simulink model "V_Cal"  (R2024b)
settings: Solver=FixedStepAuto  StartTime=0.0  StopTime=inf  RelTol=1e-3  EnableMultiTasking=on
libraries: stm32f4xxblockslib x1
settings Model: STM32="{\"AnalogInput\":[{\"ID\":\"untitled:1\"},{\"ID\":\"V_Cal:1\"}]}"  Creator=jirat  LastModifiedBy=jirat
settings OptimizationCC: DefaultParameterBehavior=Inlined  EnhancedBackFolding=on  PassReuseOutputArgsAs=Individual arguments  ZeroExternalMemoryAtStartup=off  ZeroInternalMemoryAtStartup=off  MaxStackSize=512  OptimizeBlockOrder=speed  DifferentSizesBufferReuse=on  OptimizationCustomize=off  EfficientTunableParamExpr=on
settings DebuggingCC: ParameterTunabilityLossMsg=error
settings HardwareCC: ProdBitPerPointer=32  ProdBitPerSizeT=32  ProdBitPerPtrDiffT=32  ProdLargestAtomicInteger=Long  ProdLargestAtomicFloat=Double  ProdWordSize=32  ProdLongLongMode=on  ProdHWDeviceType=ARM Compatible->ARM Cortex-M
settings SFSimCC: MATLABDynamicMemAlloc=off
settings RTWCC: Description=Embedded Coder  SystemTargetFile=ert.tlc  HardwareBoard=STM32G4xx Based  TemplateMakefile=ert_default_tmf  Toolchain=GNU Tools for ARM Embedded Processors
settings CodeAppCC: ForceParamTrailComments=on  IgnoreCustomStorageClasses=off  OperatorAnnotations=on  SimulinkDataObjDesc=on  SFDataObjDesc=on  InsertBlockDesc=on
settings ERTTargetCC: TargetLangStandard=C99 (ISO)  CodeReplacementLibrary=ARM Cortex-M  ExtModeTransport=3  ExtModeStaticAlloc=on  ExtModeStaticAllocSize=2048  ExtModeMexFile=ext_xcp  ExtModeIntrfLevel=Level2 - Open

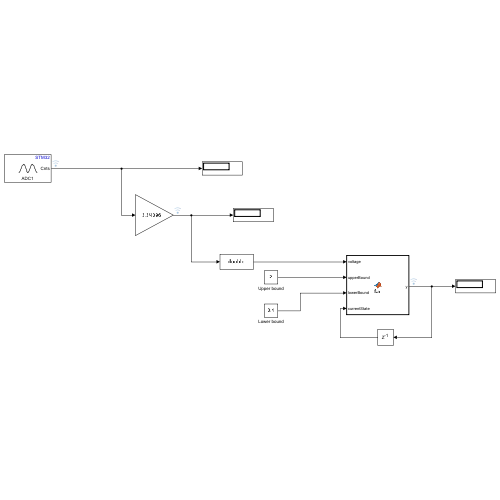
[thumbnail: Simulink's stored preview of the top-level diagram]
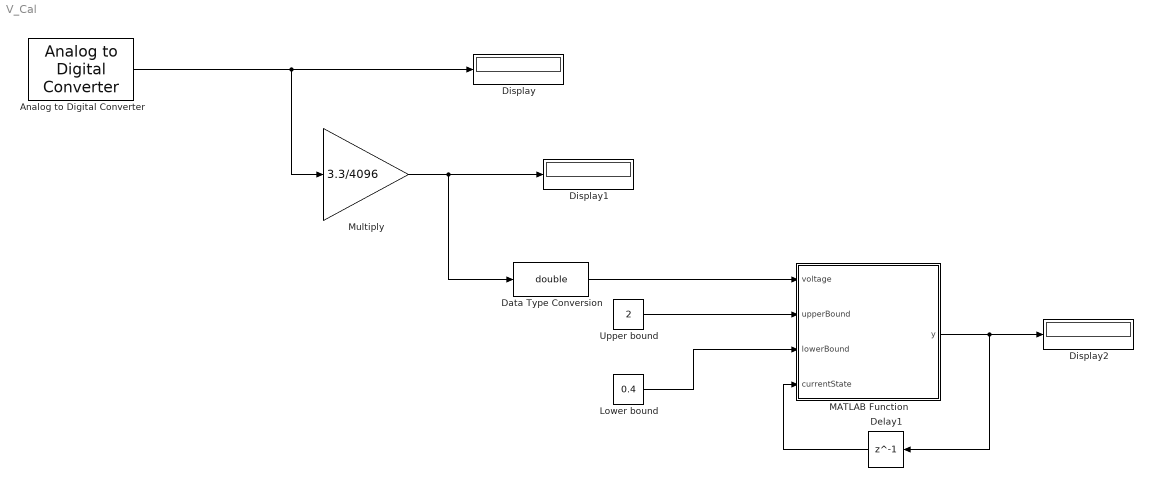
== system V_Cal ==
  Analog to Digital Converter : stm32f4xxblockslib/Analog to Digital Converter  ADCModule=ADC1  ConversionGroup=Regular  TriggerMode=Trigger and read  NumberOfConversions=1  EnableBufferConv=off  BufferLength=1  OutputStatus=off  SampleTime=-1  EnableSimPort=off  hoistedMaskSrc=ECSoC/ECSimCodegen/Analog to Digital Converter
  Data Type Conversion : DataTypeConversion  OutDataTypeStr=double  SaturateOnIntegerOverflow=off  RndMeth=Floor
  Delay1 : Delay  DelayLength=1  InputProcessing=Columns as channels (frame based)
  Display : Display
  Display1 : Display
  Display2 : Display
  Lower bound : Constant  Value=0.4
  MATLAB Function : MATLAB Function  TreatAsAtomicUnit=on
  Multiply : Gain  Gain=3.3/4096
  Upper bound : Constant  Value=2
  wires:
  Analog to Digital Converter/1 -> Multiply/1, Display/1
  Multiply/1 -> Data Type Conversion/1, Display1/1
  Upper bound/1 -> MATLAB Function/2(upperBound)
  Lower bound/1 -> MATLAB Function/3(lowerBound)
  MATLAB Function/1(y) -> Delay1/1, Display2/1
  Data Type Conversion/1 -> MATLAB Function/1(voltage)
  Delay1/1 -> MATLAB Function/4(currentState)

== matlab function V_Cal/MATLAB Function ==
  data: voltage input; y output; upperBound input; lowerBound input; currentState input
function y = fcn(voltage, upperBound, lowerBound, currentState)

    if voltage > upperBound
        y = 3.3;      
    elseif voltage < lowerBound
        y = 0;
    else
        y = currentState;
    end

end
